simulink model "ADC_RoadRunner"  (R2024b)
settings: Solver=ode23tb  StartTime=0  StopTime=20  FixedStep=0.01  RelTol=1e-3
model workspace (MAT data in the model file):
  finalint = 0
  firstWarning = 1
  originalScenarioChecksum = '114339432DE22364D47BB28FC96DC10C'
undefined symbols (not defined in the file): curvature, DefaultGear, Defined, DEND_B, DEND_S, DEND_T, direction, DiscIntNeverNeededParam, driving, dspblkCoreblockFVToolHelper, Ego, fractalcoef, gcbh, gradbp, L, Lane, LF, LR, m, MAX_BRAKE, MAX_STEER, MAX_TORQUE, maxNumActors, MCAR, MIN_BRAKE, MIN_STEER, MIN_TORQUE, n, NUMD_B, NUMD_S, NUMD_T, Pose, psi_o, R, RRdamp, sigbuilder_block, STEER_RATIO, Tdead, thetaRefs, TrackWidth, ts, Ts, User, Vdead, Velocity, WB, xRef2s, yRef2s
libraries: simulink x9, roadrunnerscenario x7, simulink_extras x4, drivingscenarioandsensors x3, sensorinslib x2, robotalgslib x1, mpcadaslib x1, drivingvehiclecontroller x1, slpidlib x1, sensorgpslib x1, mspsensorlib x1, LaneDetection x1
(part 2 of 4)

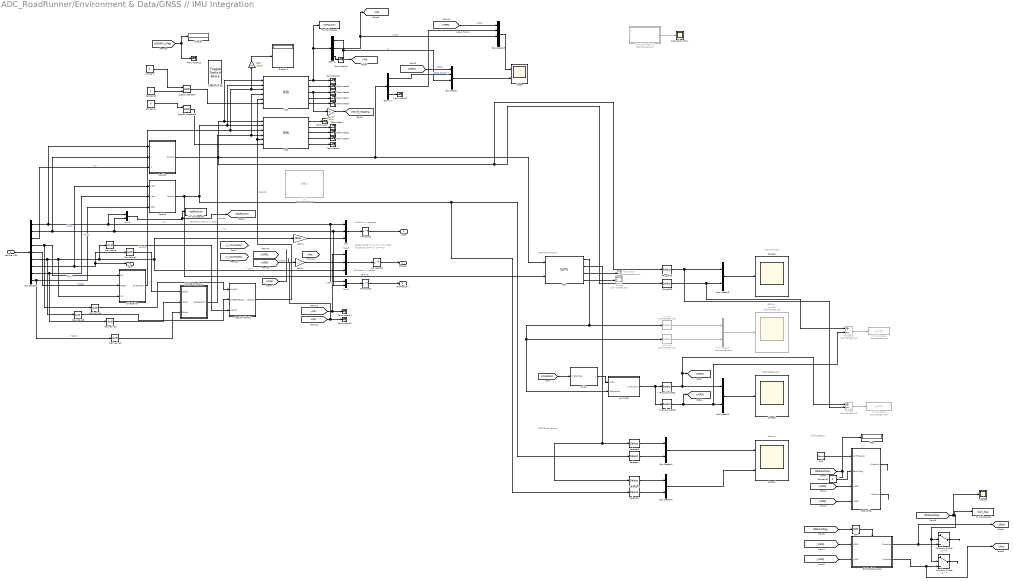
== system ADC_RoadRunner/Environment & Data/GNSS // IMU Integration ==
  note: PP Pose is in radians
  note: Drift Injection
  note: Vehicle Dynamics in NWD
  note: Cuboid to RR: Xrr = -Yc, Yrr = Xc
      | RR to Cuboid: Xc = Yrr, Yc = -Xrr
  note: Ground Truth
  note: GPS LL
  note: GPS ReferenceXY
  note: Velocity
  note: GPS Block Velocity
  note: GPS Block Position
  note: CurrPos is in degrees
  Vehicle Info : Inport
  Angular Velocity : MATLAB Function  TreatAsAtomicUnit=on  SystemSampleTime=0.05
  Bus Creator : BusCreator  Inputs=4
  Bus Creator{1..4} (4 alike) : BusCreator  Inputs=2
  Bus Creator5 : BusCreator  Inputs=4
  Bus Creator8 : BusCreator  Commented=on  Inputs=2
  Bus Selector : BusSelector  OutputSignals=InertFrm.Cg.Disp.X,InertFrm.Cg.Disp.Y,InertFrm.Cg.Disp.Z,InertFrm.Cg.Ang.phi,InertFrm.Cg.Ang.theta,InertFrm.Cg.Ang.psi,InertFrm.Cg.Vel.Xdot,InertFrm.Cg.Vel.Ydot,InertFrm.Cg.Vel.Zdot
  Constant : Constant  Value=0
  Constant1 : Constant  Value=0
  Constant2 : Constant  Value=0
  Constant3 : Constant
  Demux : Demux  Outputs=3
  Demux1 : Demux  Outputs=3
  Derivative{,1..5} (6 alike) : Derivative
  Display : Display
  Display1 : Display
  Drift : simulink/Sources/Ramp  slope=0.3  start=4  InitialOutput=0
  Flag : Display
  GPS : sensorgpslib/GPS  DispRefFrame=ENU  PositionInputFormat=Local  ReferenceLocation=[0, 0, 0]  HorizontalPositionAccuracy=0.02  VerticalPositionAccuracy=0.03  VelocityAccuracy=0.015  DecayFactor=0.9  SeedDouble=67  SimulateUsing=Code generation
  GPS Drifts : Subsystem
  GPS Packet Losses : Subsystem
  Gain : Gain  Gain=180/pi
  Gain1 : Gain  Gain=180/pi
  Gain2 : Gain  Gain=-1
  Gain3 : Gain  Gain=180/pi
  IMU : mspsensorlib/IMU  Commented=on  DispRefFrame=NED  TemperaturePort=off  Temperature=25  MagneticFieldPort=off  MagneticFieldNED=[ 27.5550, -2.4169, -16.0849 ]  MagneticFieldENU=[ -2.4169, 27.5550, 16.0849 ]  SeedDouble=67  SimulateUsing=Interpreted execution  AccelParamsMeasurementRange=Inf  AccelParamsResolution=0  AccelParamsConstantBias=[ 0, 0, 0 ]  AccelParamsAxesMisalignment=[ 100, 0, 0; 0, 100, 0; 0, 0, 100 ]  AccelParamsNoiseDensity=[ 0, 0, 0 ]  AccelParamsBiasInstability=[ 0, 0, 0 ]  AccelParamsBiasInstabilityNumerator=fractalcoef().Numerator  AccelParamsBiasInstabilityDenominator=fractalcoef().Denominator  AccelParamsRandomWalk=[ 0, 0, 0 ]  AccelParamsNoiseType=double-sided  AccelParamsTemperatureBias=[ 0, 0, 0 ]  AccelParamsTemperatureScaleFactor=[ 0, 0, 0 ]  GyroParamsMeasurementRange=Inf  GyroParamsResolution=0  GyroParamsConstantBias=[ 0, 0, 0 ]  GyroParamsAxesMisalignment=[ 100, 0, 0; 0, 100, 0; 0, 0, 100 ]  GyroParamsAccelerationBias=[ 0, 0, 0 ]  GyroParamsNoiseDensity=[ 0, 0, 0 ]  GyroParamsBiasInstability=[ 0, 0, 0 ]  GyroParamsBiasInstabilityNumerator=fractalcoef().Numerator  GyroParamsBiasInstabilityDenominator=fractalcoef().Denominator  GyroParamsRandomWalk=[ 0, 0, 0 ]  GyroParamsNoiseType=double-sided  GyroParamsTemperatureBias=[ 0, 0, 0 ]  GyroParamsTemperatureScaleFactor=[ 0, 0, 0 ]  MagParamsMeasurementRange=Inf  MagParamsResolution=0  MagParamsConstantBias=[ 0, 0, 0 ]  MagParamsAxesMisalignment=[ 100, 0, 0; 0, 100, 0; 0, 0, 100 ]  MagParamsNoiseDensity=[ 0, 0, 0 ]  MagParamsBiasInstability=[ 0, 0, 0 ]  MagParamsBiasInstabilityNumerator=fractalcoef().Numerator  MagParamsBiasInstabilityDenominator=fractalcoef().Denominator  MagParamsRandomWalk=[ 0, 0, 0 ]  MagParamsNoiseType=double-sided  MagParamsTemperatureBias=[ 0, 0, 0 ]  MagParamsTemperatureScaleFactor=[ 0, 0, 0 ]
  INS1 : sensorinslib/INS  MountingLocation=[0 0 0]  RollAccuracy=0.013  PitchAccuracy=0.013  YawAccuracy=0.07  PositionAccuracy=[0.02, 0.02, 0.03]  VelocityAccuracy=0.015  UseAccelAndAngVel=on  AccelerationAccuracy=1.18*10^-4  AngularVelocityAccuracy=0.001  TimeInput=on  PositionErrorFactor=[0.02, 0.02, 0.03]  SeedDouble=67  SimulateUsing=Code generation
      settings: LibrarySourceBlock=drivingscenarioandsensors/INS
  INS2 : sensorinslib/INS  MountingLocation=[0 0 0]  RollAccuracy=0.013  PitchAccuracy=0.013  YawAccuracy=0.07  PositionAccuracy=[0.02, 0.02, 0.03]  VelocityAccuracy=0.015  UseAccelAndAngVel=on  AccelerationAccuracy=1.18*10^-4  AngularVelocityAccuracy=0.001  TimeInput=on  PositionErrorFactor=[0.02, 0.02, 0.03]  SeedDouble=67  SimulateUsing=Code generation
      settings: LibrarySourceBlock=drivingscenarioandsensors/INS
  LLA 2 ENU : MATLAB Function  TreatAsAtomicUnit=on
  LLA_Lat : Selector  Commented=on  InputPortWidth=3  IndexOptions=Index vector (dialog)  Indices=[1]  OutputSizes=1
  LLA_Long : Selector  Commented=on  InputPortWidth=3  IndexOptions=Index vector (dialog)  Indices=[2]  OutputSizes=1
  Logical Operator : Logic  AllPortsSameDT=off  OutDataTypeStr=boolean
  Logical Operator1 : Logic  AllPortsSameDT=off  OutDataTypeStr=boolean
  MATLAB Function2 : MATLAB Function  Commented=on  TreatAsAtomicUnit=on
  MATLAB Function4 : MATLAB Function  TreatAsAtomicUnit=on  SystemSampleTime=0.05
  Mux : Mux  Inputs=3
  Mux1 : Mux  Inputs=2
  Mux2 : Mux  Inputs=3
  Mux3 : Mux  Inputs=2
  NOT : Logic  Operator=NOT  IconShape=distinctive  AllPortsSameDT=off  OutDataTypeStr=boolean
  Orientation : MATLAB Function  TreatAsAtomicUnit=on  SystemSampleTime=0.05
  Orientation Error : Scope
  Origin : MATLAB Function  TreatAsAtomicUnit=on
  Position : MATLAB Function  TreatAsAtomicUnit=on  SystemSampleTime=0.05
  Scope : Scope  NumInputPorts=2
  Scope1 : Scope  NumInputPorts=2
  Scope2 : Scope
  Scope3 : Scope
  Scope4 : Scope
  Scope5 : Scope  Commented=on
  Scope6 : Scope  Commented=on
  Selector1 : Selector  InputPortWidth=3  IndexOptions=Index vector (dialog)  Indices=[1]  OutputSizes=1
  Selector2 : Selector  InputPortWidth=3  IndexOptions=Index vector (dialog)  Indices=[2]  OutputSizes=1
  Selector3 : Selector  InputPortWidth=3  IndexOptions=Index vector (dialog)  Indices=[1]  OutputSizes=1
  Selector4 : Selector  InputPortWidth=3  IndexOptions=Index vector (dialog)  Indices=[2]  OutputSizes=1
  Subtract : Sum  Commented=on  Inputs=+-
  Subtract1 : Sum  Commented=on  Inputs=+-
  Terminator{,1..2,4..15} (15 alike) : Terminator
  Terminator3 : Terminator  Commented=on
  To Workspace : ToWorkspace  Commented=on  VariableName=x_error  SaveFormat=Structure With Time  SampleTime=-1
  To Workspace1 : ToWorkspace  Commented=on  VariableName=y_error  SaveFormat=Structure With Time  SampleTime=-1
  To Workspace2 : ToWorkspace  VariableName=insPosition  SaveFormat=Structure  SampleTime=-1
      settings: Save2DSignal=2-D array (concatenate along first dimension)
  To Workspace3 : ToWorkspace  VariableName=realPosition  SaveFormat=Structure  SampleTime=-1
      settings: Save2DSignal=2-D array (concatenate along first dimension)
  To Workspace4 : ToWorkspace  VariableName=fault_flag  SaveFormat=Structure  SampleTime=-1
      settings: Save2DSignal=2-D array (concatenate along first dimension)
  Toggle Switch : ToggleSwitchBlock
      settings: Values={{'Off', 'On'}, [0 1]}
  Transpose : Math  Operator=transpose  SignedPower=on
  Transpose1 : Math  Operator=transpose  SignedPower=on
  Transpose2 : Math  Operator=transpose  SignedPower=on
  Velocity : MATLAB Function  TreatAsAtomicUnit=on  SystemSampleTime=0.05
  XPos_GND : Selector  InputPortWidth=3  IndexOptions=Index vector (dialog)  Indices=[1]  OutputSizes=1
  XPos_Simulated : Selector  InputPortWidth=3  IndexOptions=Index vector (dialog)  Indices=[1]  OutputSizes=1
  XPosition Switch : Switch  Criteria=u2 > Threshold  SaturateOnIntegerOverflow=off  InputSameDT=off
  YPos_GND : Selector  InputPortWidth=3  IndexOptions=Index vector (dialog)  Indices=[2]  OutputSizes=1
  YPos_Simulated : Selector  InputPortWidth=3  IndexOptions=Index vector (dialog)  Indices=[2]  OutputSizes=1
  YPosition Switch : Switch  Criteria=u2 > Threshold  SaturateOnIntegerOverflow=off  InputSameDT=off
  PPpose : Outport
  pose : Outport  Port=2
  CurrPosition : Outport  Port=3
  Xdot : Outport  Port=4
  tag scope: Vehicle_Heading=global, realPosition=global, xINS=global, yINS=global, yPos=global
  wires:
  Mux/1 -> Transpose/1
  Vehicle Info/1 -> Bus Selector/1
  Gain1/1 -> Mux/3
  Transpose/1 -> pose/1
  Bus Selector/6 -> Derivative5/1, Orientation/3(psi), Derivative/1, Mux2/3, Gain1/1  "<psi>"
  Bus Selector/1 -> Position/1(X), Mux3/1, Mux1/1, Mux/1  "<X>"
  Bus Selector/2 -> Position/2(Y), Mux3/2, Mux1/2, Mux/2  "<Y>"
  Transpose2/1 -> PPpose/1
  Bus Selector/7 -> Derivative1/1, Xdot/1, Velocity/1(Xdot)  "<Xdot>"
  Bus Selector/8 -> Derivative2/1, Velocity/2(Ydot)  "<Ydot>"
  GPS/4 -> Scope5/1
  LLA_Lat/1 -> Bus Creator8/1
  XPos_GND/1 -> Subtract/2, Bus Creator3/1
  YPos_GND/1 -> Subtract1/1, Bus Creator3/2
  Bus Creator8/1 -> Scope6/1
  GPS/3 -> Terminator3/1
  [InitialPose] -> Origin/1(InitialPose)
  Position/1(Position) -> GPS/1, Demux1/1, INS2/1, INS1/1, YPos_GND/1, XPos_GND/1
  Origin/1(y) -> LLA 2 ENU/1(origin)
  Velocity/1(Velocity) -> GPS/2, INS2/2, INS1/2, Selector2/1, Selector1/1  "Velocity"
  GPS/1 -> LLA 2 ENU/2(llaPosition), LLA_Long/1, LLA_Lat/1
  GPS/2 -> Selector4/1, Selector3/1
  Bus Creator1/1 -> Scope1/1
  Selector4/1 -> Bus Creator2/1
  Bus Creator2/1 -> Scope1/2
  Selector3/1 -> Bus Creator1/1
  Selector1/1 -> Bus Creator1/2
  LLA_Long/1 -> Bus Creator8/2
  Selector2/1 -> Bus Creator2/2
  Bus Selector/3 -> Position/3(Z)  "<Z>"
  Bus Selector/9 -> Derivative3/1, Velocity/3(Zdot)  "<Zdot>"
  LLA 2 ENU/1(xyPositions) -> YPos_Simulated/1, XPos_Simulated/1
  YPos_Simulated/1 -> [yGPS], Subtract1/2, Bus Creator4/2
  Bus Creator3/1 -> Scope2/1
  Bus Creator4/1 -> Scope3/1
  XPos_Simulated/1 -> Subtract/1, [xGPS], Bus Creator4/1
  Subtract1/1 -> To Workspace1/1
  GPS Drifts/2(YPosition) -> ?
  Drift/1 -> GPS Drifts/1(Drift Signal)
  [GPSFaultFlag] -> Flag/1
  [yGPS] -> GPS Drifts/4(yGPS)
  [xGPS] -> GPS Drifts/3(xGPS)
  [GPSFaultFlag] -> NOT/1
  NOT/1 -> GPS Packet Losses/Enable
  [yGPS] -> GPS Packet Losses/2(yGPS)
  GPS Drifts/1(XPosition) -> ?
  [xGPS] -> GPS Packet Losses/1(xGPS)
  GPS Packet Losses/1(XPosition) -> [xPos], XPosition Switch/3
  GPS Packet Losses/2(yPosition) -> [yPos], YPosition Switch/3
  [GPSFaultFlag] -> Scope4/1, To Workspace4/1, YPosition Switch/2, XPosition Switch/2
  Subtract/1 -> To Workspace/1
  MATLAB Function2/1(y) -> Orientation Error/1
  Mux1/1 -> Transpose1/1
  Transpose1/1 -> CurrPosition/1
  Bus Selector/4 -> Derivative4/1, Orientation/1(phi)  "<phi>"
  Bus Selector/5 -> Orientation/2(theta)  "<theta>"
  Orientation/1(Orientation) -> INS2/3, INS1/3, Gain/1  "Velocity"
  Derivative/1 -> Angular Velocity/3(psiDot)
  Derivative1/1 -> MATLAB Function4/1(Xddot)
  Constant1/1 -> Logical Operator1/1
  INS2/2 -> Terminator1/1
  INS2/3 -> Terminator2/1
  INS2/4 -> Terminator4/1
  INS2/5 -> Terminator5/1
  INS1/5 -> Terminator6/1
  INS1/4 -> Terminator7/1
  INS1/2 -> Terminator9/1
  INS1/1 -> Terminator10/1, To Workspace2/1, Demux/1
  Derivative2/1 -> MATLAB Function4/2(Yddot)
  Derivative3/1 -> MATLAB Function4/3(Zddot)
  MATLAB Function4/1(Acceleration) -> INS2/4, INS1/4  "Velocity"
  Derivative4/1 -> Angular Velocity/1(phiDot)
  Derivative5/1 -> Angular Velocity/2(thetaDot)
  Angular Velocity/1(AngularVelocity) -> INS2/5, INS1/5  "Velocity"
  Constant3/1 -> Logical Operator/2
  [xGPS] -> Bus Creator/1  "X_GPS"
  Bus Creator/1 -> Scope/2
  [yGPS] -> Bus Creator5/1  "Y_GPS"
  Demux/2 -> Bus Creator5/3, [yINS]  "Y_INS"
  Demux1/1 -> Bus Creator/2  "GRND TRUTH_X"
  Demux/1 -> [xINS], Bus Creator/3  "X_"
  Demux1/2 -> Bus Creator5/2  "GRND TRUTH"
  Bus Creator5/1 -> Scope/1
  Demux/3 -> Terminator11/1
  Demux1/3 -> Terminator12/1
  Mux3/1 -> [realPosition], To Workspace3/1
  Mux2/1 -> Transpose2/1
  Gain2/1 -> Mux2/2
  [xINS] -> Gain2/1, Terminator15/1
  INS1/3 -> Gain3/1, Terminator8/1
  Gain/1 -> Display1/1
  Gain3/1 -> [Vehicle_Heading]
  Logical Operator1/1 -> INS2/6
  Logical Operator/1 -> INS1/6
  [GNSSFix_Flag] -> Terminator13/1, Display/1
  INS2/1 -> Terminator/1
  Constant/1 -> Logical Operator/1
  [yINS] -> Mux2/1, Terminator14/1  "Y_GPS"
  [xGPS] -> ?  "X_GPS"
  [xPos] -> ?
  XPosition Switch/1 -> ?
  YPosition Switch/1 -> ?
  Constant2/1 -> GPS Drifts/2(Fault Flag)

== system ADC_RoadRunner/Environment & Data/NWD to ENU ==
  Cuboid Pose : Inport
  Gain : Gain  Commented=through  Gain=180/pi
  Gain1 : Gain  Gain=-1
  Matrix Concatenate : Concatenate  NumInputs=3  Mode=Multidimensional array  ConcatenateDimension=2
  Selector : Selector  InputPortWidth=3  IndexOptions=Index vector (dialog)  Indices=3  OutputSizes=1
  Selector1 : Selector  InputPortWidth=3  IndexOptions=Index vector (dialog)  Indices=1  OutputSizes=1
  Selector2 : Selector  InputPortWidth=3  IndexOptions=Index vector (dialog)  Indices=2  OutputSizes=1
  RR Pose : Outport
  wires:
  Matrix Concatenate/1 -> RR Pose/1
  Selector2/1 -> Gain1/1
  Selector1/1 -> Matrix Concatenate/2
  Selector/1 -> Gain/1
  Gain1/1 -> Matrix Concatenate/1
  Gain/1 -> Matrix Concatenate/3
  Cuboid Pose/1 -> Selector1/1, Selector/1, Selector2/1

== system ADC_RoadRunner/Environment & Data/Pack Actor Pose ==
  CurrPose : Inport
  CurrSpeed : Inport  Port=2
  VehicleRuntime : Inport  Port=3
  Assign : BusAssignment  AssignedSignals=Pose,Velocity
  Bus Selector : BusSelector  OutputSignals=ActorRuntime
  Pose Generation : MATLAB Function  TreatAsAtomicUnit=on
  Selector : Selector  InputPortWidth=3  IndexOptions=Index vector (dialog)  Indices=3  OutputSizes=1
  Velocity XYZ Components : MATLAB Function  TreatAsAtomicUnit=on
  Ego Pose : Outport
  wires:
  Velocity XYZ Components/1(velocity) -> Assign/3  "Velocity"
  Pose Generation/1(currPose) -> Assign/2  "Pose"
  CurrPose/1 -> Selector/1, Pose Generation/1(pose)
  Selector/1 -> Velocity XYZ Components/1(yaw)
  CurrSpeed/1 -> Velocity XYZ Components/2(speed)
  VehicleRuntime/1 -> Bus Selector/1
  Bus Selector/1 -> Assign/1  "<ActorRuntime>"
  Assign/1 -> Ego Pose/1

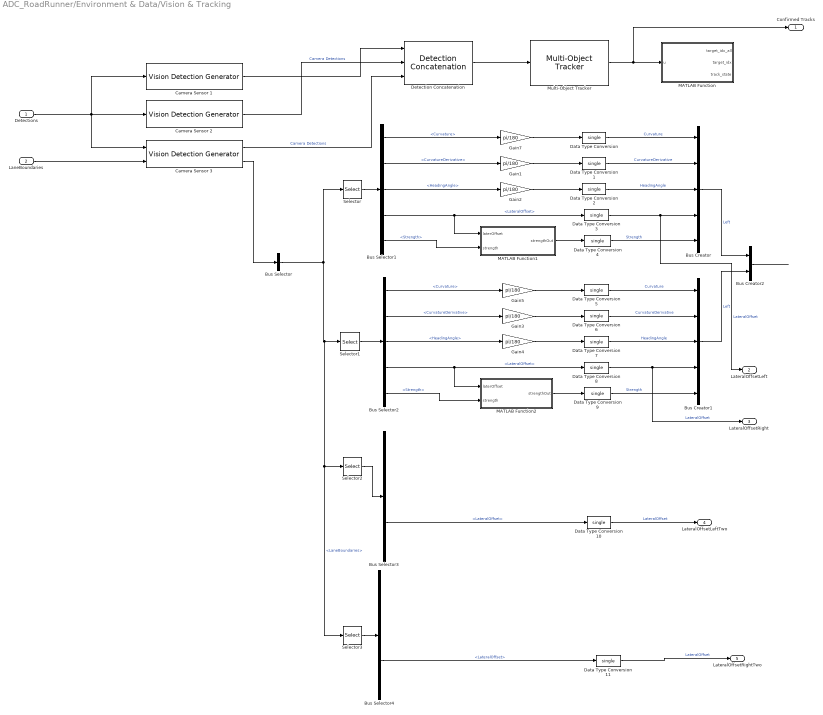
== system ADC_RoadRunner/Environment & Data/Vision & Tracking ==
  Detections : Inport
  LaneBoundaries : Inport  Port=2
  Bus Creator : BusCreator  Inputs=5
  Bus Creator1 : BusCreator  Inputs=5
  Bus Creator2 : BusCreator  Inputs=2
  Bus Selector : BusSelector  OutputSignals=LaneBoundaries
  Bus Selector{1..4} (4 alike) : BusSelector  OutputSignals=Curvature,CurvatureDerivative,HeadingAngle,LateralOffset,Strength
  Camera Sensor 1 : drivingscenarioandsensors/Vision Detection Generator  SensorIndex=1  DetectorOutput=Objects only  UpdateInterval=Ts  LaneUpdateInterval=Ts  SensorLocation=[0, 0 ]  Height=1.1  Yaw=0  Pitch=0  Roll=0  BusNameSource=Auto  BusName=BusObjectDetections  BusName2Source=Auto  BusName2=BusLaneDetections  MaxNumDetectionsSource=Property  MaxNumDetections=50  MaxNumLanesSource=Property  MaxNumLanes=30  DetectionCoordinates=Ego Cartesian  SimulateUsing=Interpreted execution  MaxRange=150  BoundingBoxAccuracy=5  ProcessNoiseIntensity=5  MaxSpeed=100  MaxAllowedOcclusion=0.5  MinObjectImageSize=[ 15, 15 ]  DetectionProbability=0.9  FalsePositivesPerImage=0.1  MinLaneImageSize=[ 20, 3 ]  LaneBoundaryAccuracy=5  HasNoise=off  InitialSeedSource=Repeatable  InitialSeed=0  UsedSeed=driving.internal.SimulinkUtilities.seedManager(gcb)  ActorProfilesSource=From Scenario Reader block  ActorProfilesParameters=driving.internal.ActorProfilesParameters  ActorProfilesExpression=struct( 'ClassID', 0, 'Length', 4.7, 'Width', 1.8, 'Height', 1.4, 'OriginOffset', [ -1.35, 0, 0 ] )  Intrinsics=driving.internal.cameraIntrinsics
  Camera Sensor 2 : drivingscenarioandsensors/Vision Detection Generator  SensorIndex=5  DetectorOutput=Objects only  UpdateInterval=Ts  LaneUpdateInterval=Ts  SensorLocation=[1.9 -0.5]  Height=2  Yaw=-45  Pitch=0  Roll=0  BusNameSource=Auto  BusName=BusObjectDetections  BusName2Source=Auto  BusName2=BusLaneDetections  MaxNumDetectionsSource=Property  MaxNumDetections=20  MaxNumLanesSource=Property  MaxNumLanes=2  DetectionCoordinates=Ego Cartesian  SimulateUsing=Code generation  MaxRange=50  BoundingBoxAccuracy=5  ProcessNoiseIntensity=5  MaxSpeed=100  MaxAllowedOcclusion=0.5  MinObjectImageSize=[5, 5]  DetectionProbability=0.9  FalsePositivesPerImage=0.1  MinLaneImageSize=[20, 5]  LaneBoundaryAccuracy=3  HasNoise=off  InitialSeedSource=Repeatable  InitialSeed=0  UsedSeed=0  ActorProfilesSource=MATLAB expression  ActorProfilesParameters=driving.internal.ActorProfilesParameters  ActorProfilesExpression=actorProfiles  Intrinsics=driving.internal.cameraIntrinsics(FocalLength=[512, 512],PrincipalPoint=[512, 384],ImageSize=[768, 1024],RadialDistortion=[0 0],TangentialDistortion=[0 0],Skew=0)
  Camera Sensor 3 : drivingscenarioandsensors/Vision Detection Generator  SensorIndex=4  DetectorOutput=Lanes and objects  UpdateInterval=Ts  LaneUpdateInterval=Ts  SensorLocation=[0, 0]  Height=1.1  Yaw=0  Pitch=0  Roll=0  BusNameSource=Auto  BusName=BusObjectDetections  BusName2Source=Auto  BusName2=BusLaneDetections  MaxNumDetectionsSource=Property  MaxNumDetections=50  MaxNumLanesSource=Property  MaxNumLanes=4  DetectionCoordinates=Ego Cartesian  SimulateUsing=Code generation  MaxRange=150  BoundingBoxAccuracy=5  ProcessNoiseIntensity=5  MaxSpeed=100  MaxAllowedOcclusion=0.5  MinObjectImageSize=[15, 15]  DetectionProbability=0.9  FalsePositivesPerImage=0.1  MinLaneImageSize=[20, 3]  LaneBoundaryAccuracy=5  HasNoise=off  InitialSeedSource=Repeatable  InitialSeed=0  UsedSeed=0  ActorProfilesSource=MATLAB expression  ActorProfilesParameters=driving.internal.ActorProfilesParameters  ActorProfilesExpression=actorProfiles  Intrinsics=driving.internal.cameraIntrinsics(FocalLength=[800, 800],PrincipalPoint=[ 320, 240 ],ImageSize=[ 480, 640 ],RadialDistortion=[0 0],TangentialDistortion=[0 0],Skew=0)
  Data Type Conversion{,1..11} (12 alike) : DataTypeConversion  OutDataTypeStr=single  SaturateOnIntegerOverflow=off  RndMeth=Floor
  Detection Concatenation : trackingutilitieslib/Detection Concatenation  NumInputs=3  BusNameSource=Auto  BusName=Detections  SimulateUsing=Code generation
  Gain{1..5,7} (6 alike) : Gain  Gain=pi/180
  MATLAB Function : MATLAB Function  TreatAsAtomicUnit=on
  MATLAB Function1 : MATLAB Function  TreatAsAtomicUnit=on
  MATLAB Function2 : MATLAB Function  TreatAsAtomicUnit=on
  Multi-Object Tracker : drivinglib/Multi-Object Tracker  TrackerIndex=uint32( 0 )  FilterInitializationFcn=helperInitSimulinkDemoFilter  AssignmentThreshold=30  ConfirmationThreshold=[ 2, 3 ]  DeletionThreshold=[ 6, 6 ]  MaxNumTracks=20  MaxNumSensors=20  OOSMHandling=Neglect  StateParametersSimulink=struct  HasStateParametersInput=off  TimeInputSource=Auto  HasCostMatrixInput=off  HasDetectableTrackIDsInput=off  BusNameSource=Auto  BusName=BusMultiObjectTracker  TentativeTracksOutputPort=off  AllTracksOutputPort=off  SimulateUsing=Interpreted execution
  Selector : Selector  InputPortWidth=4  IndexOptions=Index vector (dialog)  Indices=1  OutputSizes=1  RuntimeRangeChecks=on
  Selector1 : Selector  InputPortWidth=4  IndexOptions=Index vector (dialog)  Indices=2  OutputSizes=1
  Selector2 : Selector  InputPortWidth=4  IndexOptions=Index vector (dialog)  Indices=3  OutputSizes=1
  Selector3 : Selector  InputPortWidth=4  IndexOptions=Index vector (dialog)  Indices=4  OutputSizes=1
  Confirmed Tracks : Outport
  LateralOffsetLeft : Outport  Port=2
  LateralOffsetRight : Outport  Port=3
  LateralOffsetLeftTwo : Outport  Port=4
  LateralOffsetRightTwo : Outport  Port=5
  wires:
  Detections/1 -> Camera Sensor 1/1, Camera Sensor 2/1, Camera Sensor 3/1
  Detection Concatenation/1 -> Multi-Object Tracker/1
  Multi-Object Tracker/1 -> Confirmed Tracks/1, MATLAB Function/1(u)
  Camera Sensor 2/1 -> Detection Concatenation/2  "Camera Detections"
  Camera Sensor 3/1 -> Detection Concatenation/3  "Camera Detections"
  Camera Sensor 1/1 -> Detection Concatenation/1
  Data Type Conversion1/1 -> Bus Creator/2  "CurvatureDerivative"
  Gain1/1 -> Data Type Conversion1/1
  Data Type Conversion2/1 -> Bus Creator/3  "HeadingAngle"
  Bus Creator2/1 -> ?
  Gain7/1 -> Data Type Conversion/1
  Data Type Conversion3/1 -> LateralOffsetLeft/1, Bus Creator/4  "LateralOffset"
  Bus Selector1/5 -> MATLAB Function1/2(strength)  "<Strength>"
  Bus Selector1/1 -> Gain7/1  "<Curvature>"
  Selector/1 -> Bus Selector1/1
  Bus Creator/1 -> Bus Creator2/1  "Left"
  Bus Selector1/3 -> Gain2/1  "<HeadingAngle>"
  Data Type Conversion/1 -> Bus Creator/1  "Curvature"
  Bus Selector/1 -> Selector/1, Selector3/1, Selector2/1, Selector1/1  "<LaneBoundaries>"
  Bus Selector1/4 -> MATLAB Function1/1(laterOffset), Data Type Conversion3/1  "<LateralOffset>"
  MATLAB Function1/1(strengthOut) -> Data Type Conversion4/1
  Gain2/1 -> Data Type Conversion2/1
  Bus Selector1/2 -> Gain1/1  "<CurvatureDerivative>"
  Data Type Conversion4/1 -> Bus Creator/5  "Strength"
  MATLAB Function2/1(strengthOut) -> Data Type Conversion9/1
  Bus Creator1/1 -> Bus Creator2/2  "Left"
  Gain4/1 -> Data Type Conversion7/1
  Data Type Conversion9/1 -> Bus Creator1/5  "Strength"
  Data Type Conversion7/1 -> Bus Creator1/3  "HeadingAngle"
  Data Type Conversion5/1 -> Bus Creator1/1  "Curvature"
  Data Type Conversion6/1 -> Bus Creator1/2  "CurvatureDerivative"
  Selector1/1 -> Bus Selector2/1
  Bus Selector2/4 -> MATLAB Function2/1(laterOffset), Data Type Conversion8/1  "<LateralOffset>"
  Gain5/1 -> Data Type Conversion5/1
  Bus Selector2/3 -> Gain4/1  "<HeadingAngle>"
  Bus Selector2/1 -> Gain5/1  "<Curvature>"
  Bus Selector2/5 -> MATLAB Function2/2(strength)  "<Strength>"
  Gain3/1 -> Data Type Conversion6/1
  Bus Selector2/2 -> Gain3/1  "<CurvatureDerivative>"
  LaneBoundaries/1 -> Camera Sensor 3/2
  Camera Sensor 3/2 -> Bus Selector/1
  Data Type Conversion8/1 -> LateralOffsetRight/1, Bus Creator1/4  "LateralOffset"
  Selector2/1 -> Bus Selector3/1
  Bus Selector3/4 -> Data Type Conversion10/1  "<LateralOffset>"
  Data Type Conversion10/1 -> LateralOffsetLeftTwo/1  "LateralOffset"
  Selector3/1 -> Bus Selector4/1
  Data Type Conversion11/1 -> LateralOffsetRightTwo/1  "LateralOffset"
  Bus Selector4/4 -> Data Type Conversion11/1  "<LateralOffset>"

== system ADC_RoadRunner/Subsystem1/Reference Data1 ==
  velEgo : Inport
  xd : Inport  Port=2
  yd : Inport  Port=3
  In4 : Inport  Port=4
  LCinProgress : Inport  Port=5
  Discrete-Time Integrator : DiscreteIntegrator  SampleTime=-1  ICPrevOutput=DiscIntNeverNeededParam  ICPrevScaledInput=DiscIntNeverNeededParam
  Memory : Memory
  Memory1 : Memory
  Merge : Merge
  Merge1 : Merge
  Subsystem : Subsystem
  Subsystem1 : Subsystem
  Subsystem2 : Subsystem
  Subsystem3 : Subsystem
  Switch : Switch  Criteria=u2 ~= 0  SaturateOnIntegerOverflow=off  InputSameDT=off
  Switch Case : SwitchCase  CaseConditions={1,0}  ShowDefaultCase=off
  waypointPP : Outport
  RefPose : Outport  Port=2
  DirectionO : Outport  Port=3
  CurvatureO : Outport  Port=4
  wires:
  velEgo/1 -> Subsystem3/1(VelFdbk), Subsystem2/1(VelFdbk), Discrete-Time Integrator/1
  Subsystem2/4(WayPoints) -> Merge1/1
  Merge1/1 -> waypointPP/1
  Subsystem2/1(RefPose) -> Switch/3
  Subsystem2/2(DirectionO) -> DirectionO/1
  Merge/1 -> CurvatureO/1
  Subsystem2/3(CurvatureO) -> Merge/2
  Subsystem3/1(RefPose) -> Switch/1
  Switch Case/1 -> Subsystem3/Action
  Switch Case/2 -> Subsystem2/Action
  xd/1 -> Memory/1
  yd/1 -> Memory1/1
  Memory/1 -> Subsystem3/2(xd)
  Memory1/1 -> Subsystem3/4(yd)
  Subsystem2/5(finalint) -> Subsystem3/3(finalint)
  Subsystem/1(Out1) -> Switch/2, Switch Case/1, Subsystem1/2(enable)
  LCinProgress/1 -> Subsystem/Enable
  Discrete-Time Integrator/1 -> Subsystem1/1(Integrator)
  Subsystem1/1(Ref pose) -> RefPose/1

== system ADC_RoadRunner/Subsystem1/Subsystem ==
  function : Inport
  CurrentPose : Inport  Port=2
  MIOPos : Inport  Port=3
  Road Curvature : Inport  Port=4
  Velocity_Initial_Ego : Inport  Port=5
  MIOVel : Inport  Port=6
  laneL : Inport  Port=7
  laneR : Inport  Port=8
  V_desired : Inport  Port=9
  xref : Inport  Port=10
  yref : Inport  Port=11
  Delay : Delay  DelayLength=1
  Function-Call Subsystem : Subsystem  TreatAsAtomicUnit=on
  PathPlanner : Subsystem
  Terminator : Terminator
  To Workspace2 : ToWorkspace  VariableName=xd  SampleTime=-1
      settings: Save2DSignal=2-D array (concatenate along first dimension)
  To Workspace3 : ToWorkspace  VariableName=yd  SampleTime=-1
      settings: Save2DSignal=2-D array (concatenate along first dimension)
  Turns LC in prog off : MATLAB Function  TreatAsAtomicUnit=on
  out : Outport
  check : Outport  Port=2
  tag scope: LCinProgress=global, xd=global, yd=global
  wires:
  MIOVel/1 -> Function-Call Subsystem/5(MIOVel)
  Road Curvature/1 -> Function-Call Subsystem/3(Road Curvature)
  PathPlanner/1(out) -> out/1
  PathPlanner/2(check) -> check/1
  Velocity_Initial_Ego/1 -> Function-Call Subsystem/4(Velocity_Initial_Ego)
  V_desired/1 -> Function-Call Subsystem/6(V_desired)
  MIOPos/1 -> Function-Call Subsystem/2(MIOPos)
  Function-Call Subsystem/1(xd) -> To Workspace2/1, PathPlanner/2(xd), [xd]
  Function-Call Subsystem/2(yd) -> PathPlanner/5(yd), [yd], To Workspace3/1
  Delay/1 -> Turns LC in prog off/1(u)
  Turns LC in prog off/1(y) -> [LCinProgress]
  Function-Call Subsystem/3(LCinProgress) -> Delay/1
  CurrentPose/1 -> PathPlanner/1(CurrentPose), Function-Call Subsystem/1(EgoPosition)
  function/1 -> Function-Call Subsystem/Trigger
  laneL/1 -> Function-Call Subsystem/7(laneL)
  laneR/1 -> Function-Call Subsystem/8(laneR)
  xref/1 -> PathPlanner/3(xref)
  yref/1 -> PathPlanner/4(yref)
  PathPlanner/3(dcheck) -> Terminator/1
  [flagLC] -> PathPlanner/6(LC)

== system ADC_RoadRunner/Vehicle Dynamics/Subsystem ==
  Gain : Gain  Gain=MAX_TORQUE*0.1
  Gain1 : Gain  Gain=MIN_BRAKE*0.06
  Gain2 : Gain  Gain=MAX_STEER/4.5
  Signal Builder : Subsystem  Tag=STV Subsys  LoadFcn=sigbuilder_block('load');  StartFcn=sigbuilder_block('start');  StopFcn=sigbuilder_block('stop');  ClipboardFcn=sigbuilder_block('clipboard');  mask(Sigbuilder block){tuvar=[0:10]}
      mask help: Simulink:masks:SigbuilderBlock_MD
      mask init:
      | if ~strcmp(get_param(bdroot(gcbh),'SimulationStatus'),'stopped') tuvar = sigbuilder_block('maskInit'); end
      settings: CopyFcn=sigbuilder_block('copy');  DeleteFcn=sigbuilder_block('delete');  ModelCloseFcn=sigbuilder_block('modelClose');  PreSaveFcn=sigbuilder_block('preSave');  PauseFcn=sigbuilder_block('pause');  ContinueFcn=sigbuilder_block('continue');  NameChangeFcn=sigbuilder_block('namechange');  OpenFcn=sigbuilder_block('open',[0 30 960 455.5 ]);  CloseFcn=sigbuilder_block('close');
      mask Display: plot(0, 0, 100, 100,[2, 2, 32, 32, 2], [68, 8, 8, 68, 68],[32, 2], [38, 38], [32, 19, 2],[53, 60, 44], [32, 17, 17, 2],[16, 16, 31, 31]);txt = getActiveGroup(gcbh);text(2, 100, txt,'verticalAlignment', 'top');
  torque_cmd (Nm) : Outport
  brake_cmd (Nm) : Outport  Port=2
  steer_cmd (deg) : Outport  Port=3
  wires:
  Gain2/1 -> steer_cmd (deg)/1  "steer_cmd (deg)"
  Signal Builder/1(Normalized Torque) -> Gain/1
  Signal Builder/2(Normalized Brake) -> Gain1/1
  Signal Builder/3(Normalized Steer) -> Gain2/1  "steer_cmd (deg)"
  Gain1/1 -> brake_cmd (Nm)/1  "brake_cmd (Nm)"
  Gain/1 -> torque_cmd (Nm)/1  "torque_cmd (Nm)"

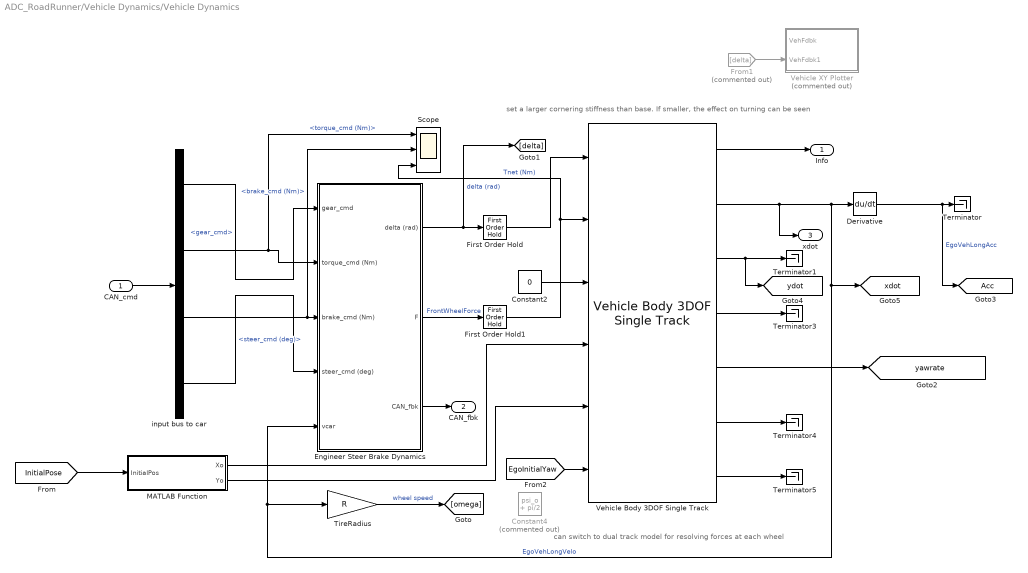
== system ADC_RoadRunner/Vehicle Dynamics/Vehicle Dynamics ==
  note: set a larger cornering stiffness than base. If smaller, the effect on turning can be seen
  note: can switch to dual track model for resolving forces at each wheel
  CAN_cmd : Inport
  Constant2 : Constant  Value=0
  Constant4 : Constant  Commented=on  Value=psi_o + pi/2
  Derivative : Derivative
  Engineer Steer Brake Dynamics : Subsystem
  First Order Hold : FirstOrderHold  ErrorTolerance=inf
  First Order Hold1 : FirstOrderHold  ErrorTolerance=inf
  From1 : From  Commented=on  GotoTag=delta
  MATLAB Function : MATLAB Function  TreatAsAtomicUnit=on
  Scope : Scope  NumInputPorts=3
  Terminator{,1,3..5} (5 alike) : Terminator
  TireRadius : Gain  Gain=R
  Vehicle Body 3DOF Single Track : autolibshared/Vehicle Body 3DOF Single Track  trackMode=Single (bicycle)  inputMode=External longitudinal forces  frontSteerMode=on  rearSteerMode=off  windMode=off  muMode=off  extFMode=off  extMMode=off  htchFMode=off  htchMMode=off  extXo=on  extpsio=on  extxdoto=off  extro=off  extYo=on  extTamb=off  extydoto=off  aMode=2  NF=2  NR=2  m=MCAR  a=LF  b=LR  h=0.35  dh=1  hh=0.2  X_o=InitPosition(1)  xdot_o=InitSpeed  CalphaMode=off  sigmaMode=on  d=0  hl=0  w=[1.4,1.4]  Cy_f=12e3*100  Cy_r=11e3*100  sigma_f=.1  sigma_r=.1  alpha_f_brk=[-.1 .1]  Cy_f_data=[-9e3 9e3]  alpha_r_brk=[-.1 .1]  Cy_r_data=[-9e3 9e3]  Y_o=-InitPosition(2)  ydot_o=0  Izz=2050  psi_o=-InitYaw/180*pi  r_o=0  Af=2  Cd=.3  Cl=.1  Cpm=.1  beta_w=[0:0.01:0.3]  Cs=[0:0.03:0.9]  Cym=[0:0.01:0.3]  Pabs=101325  Tair=273  g=9.81  mu=1  xdot_tol=.01  Fznom=5000  Fxtire_sat=7e4  Fytire_sat=7e4  longOff=0  latOff=0  vertOff=0  wrapAng=off
  Vehicle XY Plotter : Subsystem  Commented=on  mask(Vehicle XY Plotter){a=LF, b=LR, w=TrackWidth, bufferSize=1024, pltDT=.1}
      mask prompts: a "Distance to front axle from CG, a [m]:"; b "Distance to rear axle from CG, b [m]:"; w "Track width, w [m]:"; bufferSize "Path buffer sampe size, bufferSize []:"; pltDT "Plot update rate, pltDT [s]:"
      mask help: This block will display a MATLAB figure which indicates the vehicle path, current position and heading velocity.
      mask TypeOptions a: Vehicle XY Plotter/a
      mask TypeOptions b: Vehicle XY Plotter/b
      mask TypeOptions w: Vehicle XY Plotter/w
      mask TypeOptions bufferSize: Vehicle XY Plotter/bufferSize
  input bus to car : BusSelector  OutputSignals=gear_cmd,torque_cmd (Nm),brake_cmd (Nm),steer_cmd (deg)
  Info : Outport
  CAN_fbk : Outport  Port=2  VectorParamsAs1DForOutWhenUnconnected=off
  xdot : Outport  Port=3
  tag scope: Acc=global, xdot=global, yawrate=global, ydot=global
  wires:
  TireRadius/1 -> [omega]  "wheel speed"
  Vehicle Body 3DOF Single Track/1 -> Info/1
  From1/1 -> Vehicle XY Plotter/2(VehFdbk1)
  input bus to car/1 -> Engineer Steer Brake Dynamics/1(gear_cmd)  "<gear_cmd>"
  input bus to car/3 -> Scope/2, Engineer Steer Brake Dynamics/3(brake_cmd (Nm))  "<brake_cmd (Nm)>"
  Engineer Steer Brake Dynamics/1(delta (rad)) -> [delta], First Order Hold/1  "delta (rad)"
  input bus to car/2 -> Scope/1, Engineer Steer Brake Dynamics/2(torque_cmd (Nm))  "<torque_cmd (Nm)>"
  input bus to car/4 -> Engineer Steer Brake Dynamics/4(steer_cmd (deg))  "<steer_cmd (deg)>"
  Engineer Steer Brake Dynamics/3(CAN_fbk) -> CAN_fbk/1
  CAN_cmd/1 -> input bus to car/1
  Constant2/1 -> Vehicle Body 3DOF Single Track/3
  Engineer Steer Brake Dynamics/2(F) -> First Order Hold1/1  "FrontWheelForce"
  First Order Hold/1 -> Vehicle Body 3DOF Single Track/1
  Vehicle Body 3DOF Single Track/2 -> [xdot], Engineer Steer Brake Dynamics/5(vcar), TireRadius/1, Derivative/1, xdot/1  "EgoVehLongVelo"
  Vehicle Body 3DOF Single Track/3 -> [ydot], Terminator1/1
  Vehicle Body 3DOF Single Track/4 -> Terminator3/1
  Vehicle Body 3DOF Single Track/5 -> [yawrate]
  Vehicle Body 3DOF Single Track/6 -> Terminator4/1
  Vehicle Body 3DOF Single Track/7 -> Terminator5/1
  Derivative/1 -> [Acc], Terminator/1  "EgoVehLongAcc"
  First Order Hold1/1 -> Scope/3, Vehicle Body 3DOF Single Track/2  "Tnet (Nm)"
  MATLAB Function/1(Xo) -> Vehicle Body 3DOF Single Track/4
  MATLAB Function/2(Yo) -> Vehicle Body 3DOF Single Track/5
  [InitialPose] -> MATLAB Function/1(InitialPos)
  [EgoInitialYaw] -> Vehicle Body 3DOF Single Track/6

== system ADC_RoadRunner/Controllers/Lateral Controllers1/Pure Pursuit Controller1 ==
  note: The subsystem implements a Pure Pursuit controller. The "Pure Pursuit" block calculates the target direction and the "Wheel Steering Angle Formulation" block calculates the wheel steering angle.
  Pose : Inport
  Waypoints : Inport  Port=2
  Pure Pursuit : robotalgslib/Pure Pursuit  DesiredLinearVelocityPort=off  DesiredLinearVelocity=0.1  MaxAngularVelocity=1.0  LookaheadDistancePort=off  LookaheadDistance=10  TargetDirPort=on  SimulateUsing=Interpreted execution
  Terminator6 : Terminator
  Terminator7 : Terminator
  Wheel Steering Angle Formulation : Subsystem  mask{L=L, ld=10}
      mask prompts: L "Bicycle length"; ld "Lookahead distance"
      mask TypeOptions L: Bicycle length/Value
      mask TypeOptions ld: Lookahead distance/Value
      mask Display:
      | image("GeometryMask.png")
      | port_label('input', 1, 'alpha')
      | port_label('output', 1, 'delta')
  delta : Outport
  wires:
  Wheel Steering Angle Formulation/1(Al) -> delta/1
  Pure Pursuit/3 -> Wheel Steering Angle Formulation/1(alpha)
  Pure Pursuit/2 -> Terminator7/1
  Pose/1 -> Pure Pursuit/1
  Pure Pursuit/1 -> Terminator6/1
  Waypoints/1 -> Pure Pursuit/2

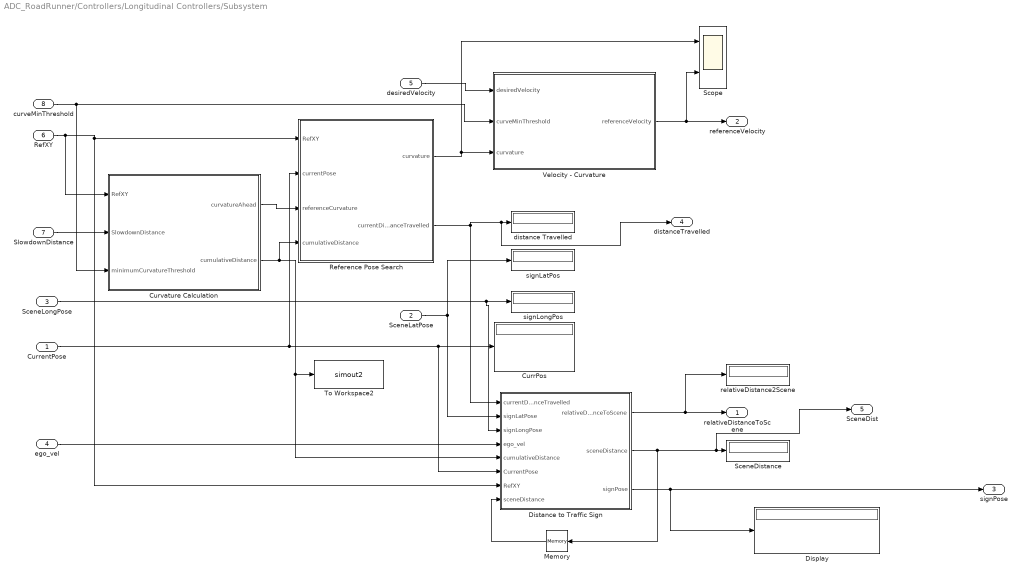
== system ADC_RoadRunner/Controllers/Longitudinal Controllers/Subsystem ==
  CurrentPose : Inport
  SceneLatPose : Inport  Port=2
  SceneLongPose : Inport  Port=3
  ego_vel : Inport  Port=4
  desiredVelocity : Inport  Port=5
  RefXY : Inport  Port=6
  SlowdownDistance : Inport  Port=7
  curveMinThreshold : Inport  Port=8
  CurrPos : Display
  Curvature Calculation : MATLAB Function  TreatAsAtomicUnit=on
  Display : Display
  Distance to Traffic Sign : MATLAB Function  TreatAsAtomicUnit=on
  Memory : Memory  InitialCondition=300
  Reference Pose Search : MATLAB Function  TreatAsAtomicUnit=on
  SceneDistance : Display
  Scope : Scope  NumInputPorts=2
  To Workspace2 : ToWorkspace  VariableName=simout2  SaveFormat=Structure  SampleTime=-1
      settings: Save2DSignal=2-D array (concatenate along first dimension)
  Velocity - Curvature : MATLAB Function  TreatAsAtomicUnit=on
  distance Travelled : Display
  relativeDistance2Scene : Display
  signLatPos : Display
  signLongPos : Display
  relativeDistanceToScene : Outport
  referenceVelocity : Outport  Port=2
  signPose : Outport  Port=3
  distanceTravelled : Outport  Port=4
  SceneDist : Outport  Port=5
  wires:
  Distance to Traffic Sign/3(signPose) -> Display/1, signPose/1
  Distance to Traffic Sign/2(sceneDistance) -> SceneDist/1, SceneDistance/1, Memory/1
  Distance to Traffic Sign/1(relativeDistanceToScene) -> relativeDistanceToScene/1, relativeDistance2Scene/1
  Velocity - Curvature/1(referenceVelocity) -> Scope/2, referenceVelocity/1
  ego_vel/1 -> Distance to Traffic Sign/4(ego_vel)
  CurrentPose/1 -> Reference Pose Search/2(currentPose), Distance to Traffic Sign/6(CurrentPose), CurrPos/1
  Curvature Calculation/1(curvatureAhead) -> Reference Pose Search/3(referenceCurvature)
  Memory/1 -> Distance to Traffic Sign/8("sceneDistance ")
  Curvature Calculation/2(cumulativeDistance) -> Reference Pose Search/4(cumulativeDistance), To Workspace2/1, Distance to Traffic Sign/5(cumulativeDistance)
  desiredVelocity/1 -> Velocity - Curvature/1(desiredVelocity)
  Reference Pose Search/1(curvature) -> Scope/1, Velocity - Curvature/3(curvature)
  SceneLongPose/1 -> Distance to Traffic Sign/3(signLongPose), signLongPos/1
  curveMinThreshold/1 -> Curvature Calculation/3(minimumCurvatureThreshold), Velocity - Curvature/2(curveMinThreshold)
  SlowdownDistance/1 -> Curvature Calculation/2(SlowdownDistance)
  Reference Pose Search/2(currentDistanceTravelled) -> distanceTravelled/1, distance Travelled/1, Distance to Traffic Sign/1(currentDistanceTravelled)
  SceneLatPose/1 -> signLatPos/1, Distance to Traffic Sign/2(signLatPose)
  RefXY/1 -> Reference Pose Search/1(RefXY), Distance to Traffic Sign/7(RefXY), Curvature Calculation/1(RefXY)

== system ADC_RoadRunner/Controllers/Subsystem2/Acceleration to Torque ==
  acc_cmd : Inport
  decc_cmd : Inport  Port=2
  Brake Saturation : Saturate  UpperLimit=MAX_BRAKE  LowerLimit=MIN_BRAKE
  Constant : Constant  Value=0
  Gain2 : Gain  Gain=1/(400*2)
  Subsystem2 : Subsystem
  Switch : Switch  Criteria=u2 > Threshold  Threshold=500  SaturateOnIntegerOverflow=off  InputSameDT=off
  Switch1 : Switch  Criteria=u2 > Threshold  Threshold=-500  SaturateOnIntegerOverflow=off  InputSameDT=off
  Throttle Saturation : Saturate  UpperLimit=MAX_TORQUE  LowerLimit=MIN_TORQUE
  second-order low-pass brake model1 : DiscreteTransferFcn  Commented=through  Numerator=DEND_B  Denominator=NUMD_B  SampleTime=ts
  second-order low-pass torque model : DiscreteTransferFcn  Commented=through  Numerator=DEND_T  Denominator=NUMD_T  SampleTime=ts
  torque_cm : Outport
  brake_cm : Outport  Port=2
  ActualAccel : Outport  Port=3
  wires:
  Subsystem2/1(T_eng_cmd) -> second-order low-pass torque model/1
  acc_cmd/1 -> Subsystem2/1(acc_cmd)
  second-order low-pass brake model1/1 -> Brake Saturation/1
  Subsystem2/2(brake_cmd) -> second-order low-pass brake model1/1
  decc_cmd/1 -> Subsystem2/2(decc_cmd)
  second-order low-pass torque model/1 -> Throttle Saturation/1
  Throttle Saturation/1 -> Switch/2, Switch/1
  Switch/1 -> Gain2/1, torque_cm/1
  Brake Saturation/1 -> Switch1/2, Switch1/3
  Switch1/1 -> brake_cm/1
  Constant/1 -> Switch/3, Switch1/1
  Gain2/1 -> ActualAccel/1

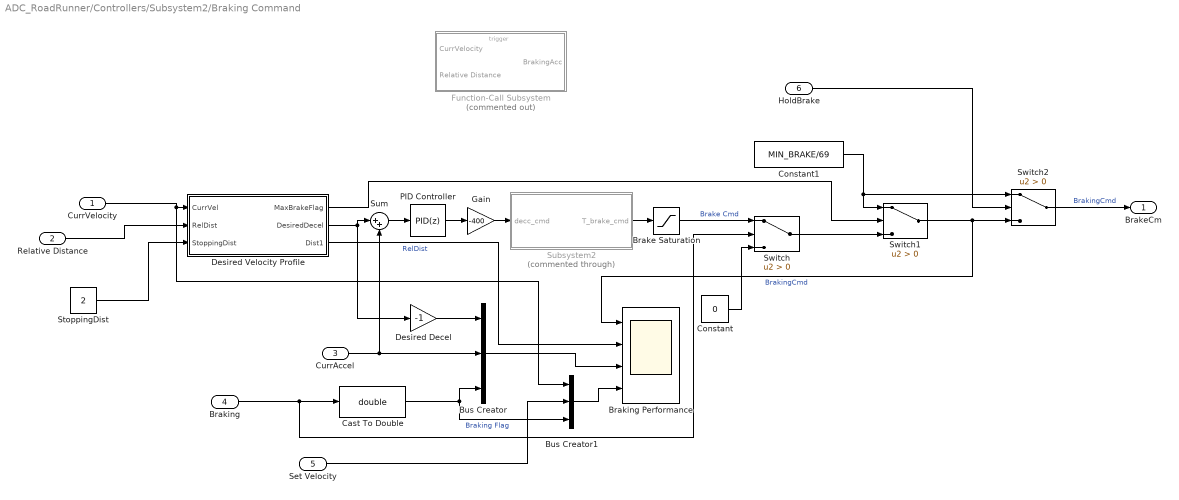
== system ADC_RoadRunner/Controllers/Subsystem2/Braking Command ==
  CurrVelocity : Inport
  Relative Distance : Inport  Port=2
  CurrAccel : Inport  Port=3
  "Braking " : Inport  Port=4
  Set Velocity : Inport  Port=5
  HoldBrake : Inport  Port=6
  Brake Saturation : Saturate  UpperLimit=MAX_BRAKE  LowerLimit=MIN_BRAKE
  Braking Performance : Scope  NumInputPorts=4
  Bus Creator : BusCreator  Inputs=3
  Bus Creator1 : BusCreator  Inputs=3
  Cast To Double : DataTypeConversion  OutDataTypeStr=double  SaturateOnIntegerOverflow=off  RndMeth=Floor
  Constant : Constant  Value=0
  Constant1 : Constant  Value=MIN_BRAKE/69
  Desired Decel : Gain  Gain=-1
  Desired Velocity Profile : MATLAB Function  TreatAsAtomicUnit=on
  Function-Call Subsystem : Subsystem  Commented=on  TreatAsAtomicUnit=on
  Gain : Gain  Gain=-400
  PID Controller : slpidlib/PID Controller  Controller=PID  Form=Parallel  TimeDomain=Discrete-time  UseExternalTs=off  SampleTime=-1  IntegratorMethod=Forward Euler  FilterMethod=Forward Euler  ControllerParametersSource=internal  P=0.05*20  I=0.01*10  UseKiTs=off  D=0  UseExternalDerivativeSource=off  N=100  UseFilter=on  TunerSelectOption=Transfer Function Based (PID Tuner App)  InitialConditionSource=internal  InitialConditionForIntegrator=0  InitialConditionForFilter=0  DifferentiatorICPrevScaledInput=0  ExternalReset=none  TrackingMode=off  Kt=1  LimitOutput=off  SatLimitsSource=internal  UpperSaturationLimit=inf  LowerSaturationLimit=-inf  LinearizeAsGain=on  AntiWindupMode=none  Kb=1  LimitIntegrator=off  UpperIntegratorSaturationLimit=inf  LowerIntegratorSaturationLimit=-inf  POutMin=[]  POutMax=[]  IOutMin=[]  IOutMax=[]  DOutMin=[]  DOutMax=[]  NOutMin=[]  NOutMax=[]  SumOutMin=[]  SumOutMax=[]  SaturationOutMin=[]  SaturationOutMax=[]  PParamMin=[]  PParamMax=[]  IParamMin=[]  IParamMax=[]  DParamMin=[]  DParamMax=[]  NParamMin=[]  NParamMax=[]  KbParamMin=[]  KbParamMax=[]  KtParamMin=[]  KtParamMax=[]  KbOutMin=[]  KbOutMax=[]  KtOutMin=[]  KtOutMax=[]  IntegratorOutMin=[]  IntegratorOutMax=[]  FilterOutMin=[]  FilterOutMax=[]  SumI1OutMin=[]  SumI1OutMax=[]  SumI2OutMin=[]  SumI2OutMax=[]  SumI3OutMin=[]  SumI3OutMax=[]  SumI4OutMin=[]  SumI4OutMax=[]  SumDOutMin=[]  SumDOutMax=[]  DifferentiatorOutMin=[]  DifferentiatorOutMax=[]  FilterDiffOutCoefMin=[]  FilterDiffOutCoefMax=[]  ReciprocalOutMin=[]  ReciprocalOutMax=[]  SumDenOutMin=[]  SumDenOutMax=[]  SumNumOutMin=[]  SumNumOutMax=[]  DivideOutMin=[]  DivideOutMax=[]  UdiffTsProdOutMin=[]  UdiffTsProdOutMax=[]  NTsProdOutMin=[]  NTsProdOutMax=[]  UintegralTsProdOutMin=[]  UintegralTsProdOutMax=[]  UngainTsProdOutMin=[]  UngainTsProdOutMax=[]  ClampingZeroOutDataTypeStr=Inherit: Inherit via back propagation  ClampingZeroOutMin=[]  ClampingZeroOutMax=[]  FilterDenConstantOutDataTypeStr=Inherit: Inherit via back propagation  FilterDenConstantOutMin=[]  FilterDenConstantOutMax=[]  PCopyOutDataTypeStr=Inherit: Inherit via back propagation  PCopyOutMin=[]  PCopyOutMax=[]  NCopyOutDataTypeStr=Inherit: Inherit via back propagation  NCopyOutMin=[]  NCopyOutMax=[]  IntegratorContinuousStateAttributes=''  IntegratorStateMustResolveToSignalObject=off  IntegratorRTWStateStorageClass=Auto  FilterContinuousStateAttributes=''  FilterStateMustResolveToSignalObject=off  FilterRTWStateStorageClass=Auto  ParallelPVariant=InternalParameters  IdealPVariant=Disabled  IVariant=InternalParameters  DVariant=InternalParameters  IntegratorVariant=Discrete  SatVariant=Disabled  AWVariant=Passthrough  PCopyVariant=Disabled  TRVariant=Disabled  FdbkBlocksVariant=Forward  IdealPFdbkVariant=Disabled  SatFdbkVariant=Disabled  DerivativeFilterVariant=ForwardEulerFilter  NVariant=InternalParameters  NCopyVariant=Disabled  FilterICVariant=InternalICsFilter  IntegratorICVariant=InternalICs  ExternalResetVariant=Disabled  TRSumVariant=Passthrough  SumFdbkVariant=Disabled  SumVariant=Sum_PID  TsampFilterVariant=InternalTs  TsampNgainVariant=Passthrough  TsampIntegralVariant=Disabled_SignalSpec  ExternalSaturationOutDataTypeStr=Inherit: Same as second input  DerivativeSourceVariant=ErrorSignal  PreIntVariant=InternalPreInt
  StoppingDist : Constant  Value=2
  Subsystem2 : Subsystem  Commented=through
  Sum : Sum  Inputs=|++
  Switch : Switch  Criteria=u2 > Threshold  SaturateOnIntegerOverflow=off  InputSameDT=off
  Switch1 : Switch  Criteria=u2 > Threshold  SaturateOnIntegerOverflow=off  InputSameDT=off
  Switch2 : Switch  Criteria=u2 > Threshold  SaturateOnIntegerOverflow=off  InputSameDT=off
  BrakeCm : Outport
  wires:
  PID Controller/1 -> Gain/1
  Relative Distance/1 -> Desired Velocity Profile/2(RelDist)
  CurrVelocity/1 -> Bus Creator1/1, Desired Velocity Profile/1(CurrVel)
  Sum/1 -> PID Controller/1
  Subsystem2/1(T_brake_cmd) -> Brake Saturation/1
  "Braking "/1 -> Cast To Double/1, Switch/2
  Brake Saturation/1 -> Switch/1  "Brake Cmd"
  CurrAccel/1 -> Bus Creator/2, Sum/2
  Gain/1 -> Subsystem2/1(decc_cmd)
  Desired Decel/1 -> Bus Creator/1
  Constant/1 -> Switch/3
  Switch1/1 -> Switch2/3, Braking Performance/1  "BrakingCmd"
  Bus Creator/1 -> Braking Performance/3
  Cast To Double/1 -> Bus Creator1/3, Bus Creator/3  "Braking Flag"
  Desired Velocity Profile/3(Dist1) -> Braking Performance/2  "RelDist"
  Switch/1 -> Switch1/3
  Constant1/1 -> Switch2/1, Switch1/1
  Desired Velocity Profile/1(MaxBrakeFlag) -> Switch1/2
  Bus Creator1/1 -> Braking Performance/4
  Set Velocity/1 -> Bus Creator1/2
  StoppingDist/1 -> Desired Velocity Profile/3(StoppingDist)
  HoldBrake/1 -> Switch2/2
  Switch2/1 -> BrakeCm/1  "BrakingCmd"
  Desired Velocity Profile/2(DesiredDecel) -> Sum/1, Desired Decel/1

== system ADC_RoadRunner/Environment & Data/GNSS // IMU Integration/GPS Drifts ==
  Drift Signal : Inport
  Fault Flag : Inport  Port=2
  xGPS : Inport  Port=3
  yGPS : Inport  Port=4
  Add : Sum
  Add1 : Sum
  Bus Creator : BusCreator  Inputs=2
  Bus Creator1 : BusCreator  Inputs=2
  Constant : Constant  Value=0
  Scope : Scope
  Switch : Switch  Criteria=u2 > Threshold  SaturateOnIntegerOverflow=off  InputSameDT=off
  Switch1 : Switch  Criteria=u2 > Threshold  SaturateOnIntegerOverflow=off  InputSameDT=off
  yPos Drift : Scope
  XPosition : Outport
  YPosition : Outport  Port=2
  wires:
  Bus Creator1/1 -> Scope/1
  Drift Signal/1 -> Add1/1, Add/1
  Switch1/1 -> YPosition/1
  xGPS/1 -> Switch/3, Bus Creator1/1, Add/2
  Add1/1 -> Switch1/1, Bus Creator/2
  Fault Flag/1 -> Switch1/2, Switch/2
  Add/1 -> Bus Creator1/2, Switch/1
  yGPS/1 -> Bus Creator/1, Switch1/3, Add1/2
  Switch/1 -> XPosition/1
  Bus Creator/1 -> yPos Drift/1

== system ADC_RoadRunner/Environment & Data/GNSS // IMU Integration/GPS Packet Losses ==
  xGPS : Inport
  yGPS : Inport  Port=2
  Enable : EnablePort
  XPosition : Outport
  yPosition : Outport  Port=2
  wires:
  xGPS/1 -> XPosition/1
  yGPS/1 -> yPosition/1

== system ADC_RoadRunner/Subsystem1/Reference Data1/Subsystem ==
  In1 : Inport
  Enable : EnablePort
  Step : Step
  Step1 : Step  Time=10
  Sum : Sum  Inputs=|+-
  Out1 : Outport
  wires:
  Sum/1 -> Out1/1
  Step/1 -> Sum/1
  Step1/1 -> Sum/2

== system ADC_RoadRunner/Subsystem1/Reference Data1/Subsystem1 ==
  Integrator : Inport
  enable : Inport  Port=2
  Display : Display
  Subsystem2 : Subsystem
  Subsystem3 : Subsystem
  Switch : Switch  Threshold=1  SaturateOnIntegerOverflow=off  InputSameDT=off
  Ref pose : Outport
  wires:
  enable/1 -> Switch/2
  Integrator/1 -> Subsystem2/1(Integrator), Subsystem3/2(integrator)
  Subsystem2/1(RefPose) -> Display/1, Switch/3
  Subsystem3/1(RefPose) -> Switch/1
  Switch/1 -> Ref pose/1

== system ADC_RoadRunner/Subsystem1/Reference Data1/Subsystem2 ==
  VelFdbk : Inport
  Action Port : ActionPort
  Subsystem : Subsystem
  RefPose : Outport
  DirectionO : Outport  Port=2
  CurvatureO : Outport  Port=3
  WayPoints : Outport  Port=4
  finalint : Outport  Port=5
  wires:
  Subsystem/1(Out1) -> WayPoints/1
  Subsystem/4(DirectionO) -> DirectionO/1
  VelFdbk/1 -> Subsystem/1(In1)
  Subsystem/2(Out2) -> RefPose/1
  Subsystem/3(CurvatureO) -> CurvatureO/1
  Subsystem/5(finalint) -> finalint/1

== system ADC_RoadRunner/Subsystem1/Reference Data1/Subsystem3 ==
  VelFdbk : Inport
  xd : Inport  Port=2
  finalint : Inport  Port=3
  yd : Inport  Port=4
  Action Port : ActionPort
  Subsystem : Subsystem
  RefPose : Outport
  DirectionO : Outport  Port=2
  CurvatureO : Outport  Port=3
  WayPoints : Outport  Port=4
  wires:
  Subsystem/1(Out1) -> WayPoints/1
  Subsystem/4(DirectionO) -> DirectionO/1
  VelFdbk/1 -> Subsystem/1(In1)
  Subsystem/2(Out2) -> RefPose/1
  Subsystem/3(CurvatureO) -> CurvatureO/1
  xd/1 -> Subsystem/2(xd)
  yd/1 -> Subsystem/4(yd)
  finalint/1 -> Subsystem/3(finalint)

== system ADC_RoadRunner/Subsystem1/Subsystem/Function-Call Subsystem ==
  note: put multipler just to change sign to check
  EgoPosition : Inport
  MIOPos : Inport  Port=2
  Road Curvature : Inport  Port=3
  Velocity_Initial_Ego : Inport  Port=4
  MIOVel : Inport  Port=5
  V_desired : Inport  Port=6
  laneL : Inport  Port=7
  laneR : Inport  Port=8
  function : TriggerPort  VariantControl=(inherit)  ShowOutputPort=on
  MATLAB Function1 : MATLAB Function  Commented=on  TreatAsAtomicUnit=on
  MATLAB Function2 : MATLAB Function  TreatAsAtomicUnit=on
  Multiply : Gain  Commented=through  Gain=-1
  Multiply1 : Gain  Gain=-1
  Scope : Scope  NumInputPorts=2
  xd : Outport  InitialOutput=zeros(99,1)
  yd : Outport  Port=2  InitialOutput=zeros(99,1)
  LCinProgress : Outport  Port=3  InitialOutput=0
  wires:
  EgoPosition/1 -> MATLAB Function2/1(EgoPosition), MATLAB Function1/1(EgoPosition)
  MIOPos/1 -> MATLAB Function2/2(MIOPos), MATLAB Function1/2(MIOPos)
  Road Curvature/1 -> MATLAB Function2/3(curvature), MATLAB Function1/3(curvature)
  MIOVel/1 -> MATLAB Function2/4(MIOVel), MATLAB Function1/4(MIOVel)
  Velocity_Initial_Ego/1 -> MATLAB Function2/5(V_i), MATLAB Function1/5(V_i)
  ? -> Scope/1
  ? -> Multiply/1, Scope/2
  V_desired/1 -> MATLAB Function2/8(V_desired), MATLAB Function1/8(V_desired)
  laneL/1 -> MATLAB Function2/6(laneL), MATLAB Function1/6(laneL)
  laneR/1 -> MATLAB Function2/7(laneR), MATLAB Function1/7(laneR)
  Multiply1/1 -> yd/1
  MATLAB Function2/1(xd) -> xd/1
  MATLAB Function2/2(yd) -> Multiply1/1
  MATLAB Function2/3(LCinProgress) -> LCinProgress/1

== system ADC_RoadRunner/Subsystem1/Subsystem/PathPlanner ==
  note: The Path Planning module takes in Trajector generated during Lane change
      | and merges it with current trajectory.
      |
      |
      | If Lane change takes place: Planning module will only work on straight roads.
      |
      | if Lane change doesnt take place: Planning module will work anyway
  CurrentPose : Inport
  xd : Inport  Port=2
  xref : Inport  Port=3
  yref : Inport  Port=4
  yd : Inport  Port=5
  LC : Inport  Port=6
  Cast To Boolean : DataTypeConversion  OutDataTypeStr=boolean  SaturateOnIntegerOverflow=off  RndMeth=Floor
  Delay1 : Delay  DelayLength=1
  Delay2 : Delay  DelayLength=1
  Demux : Demux  Outputs=3
  MATLAB Function3 : MATLAB Function  TreatAsAtomicUnit=on
  MATLAB Function4 : MATLAB Function  TreatAsAtomicUnit=on
  Rate Transition : RateTransition
  Terminator : Terminator
  out : Outport
  check : Outport  Port=2
  dcheck : Outport  Port=3
  wires:
  MATLAB Function3/3(dcheck) -> dcheck/1
  MATLAB Function4/1(Distance) -> Delay1/1
  yd/1 -> MATLAB Function3/4(yd)
  Delay1/1 -> MATLAB Function3/7(d2f)
  CurrentPose/1 -> Demux/1, MATLAB Function4/2(CurrentPose)
  MATLAB Function4/2(point) -> Terminator/1
  MATLAB Function3/1(out) -> MATLAB Function4/1(output), out/1
  xd/1 -> MATLAB Function3/3(xd)
  LC/1 -> MATLAB Function3/5(LC), Delay2/1
  Delay2/1 -> Rate Transition/1
  Demux/2 -> MATLAB Function3/6(current_pos)
  Cast To Boolean/1 -> check/1
  MATLAB Function3/2(check) -> Cast To Boolean/1
  xref/1 -> MATLAB Function3/1(Xref)
  yref/1 -> MATLAB Function3/2(Yref)
